simulink model "Exercitiul_2"  (R2021b)
settings: Solver=VariableStepAuto  StartTime=0.0  StopTime=10.0  RelTol=1e-3
libraries: simulink x1
settings Model: Creator=Petrisor  LastModifiedBy=Petrisor

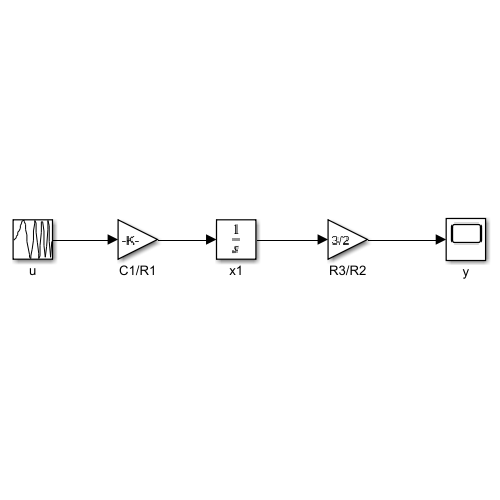
[thumbnail: Simulink's stored preview of the top-level diagram]
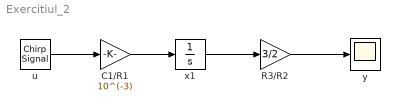
== system Exercitiul_2 ==
  C1/R1 : Gain  Gain=10^(-3)
  R3/R2 : Gain  Gain=3/2
  u : simulink/Sources/Chirp Signal  f1=0.01  T=10  f2=10^10
  x1 : Integrator
  y : Scope
  wires:
  R3/R2/1 -> y/1
  x1/1 -> R3/R2/1
  C1/R1/1 -> x1/1
  u/1 -> C1/R1/1
